simulink model "Mensajes"  (R2023a)
settings: Solver=VariableStepAuto  StartTime=0.0  StopTime=10.0  RelTol=1e-3
settings Model: Creator=santi  LastModifiedBy=santi

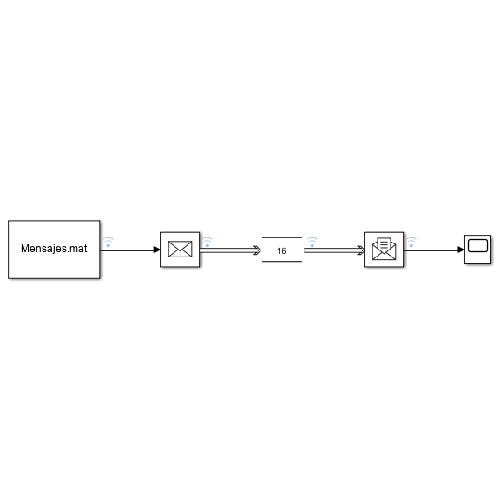
[thumbnail: Simulink's stored preview of the top-level diagram]
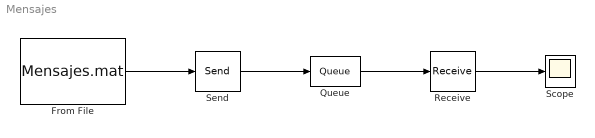
== system Mensajes ==
  From File : FromFile  FileName=Mensajes.mat  SampleTime=0
  Queue : Queue  InputPortMessageModes=m  OutputPortMessageModes=m  OverwriteOldest=on  Capacity=16
  Receive : Receive  InputPortMessageModes=m
  Scope : Scope
  Send : Send  OutputPortMessageModes=m
  wires:
  From File/1 -> Send/1
  Send/1 -> Queue/1
  Queue/1 -> Receive/1
  Receive/1 -> Scope/1
